simulink model "Bruening_4t_showshuffle"  (R2015a)
settings: Solver=ode4  SolverMode=MultiTasking  StartTime=0.0  StopTime=inf  FixedStep=BKIN_STEP_TIME  RelTol=1e-3
StartFcn:
  |  warndlg('Dexterit-E models cannot run under simulation. Please compile your model and run it from within Dexterit-E.');set_param(bdroot,'SimulationCommand','stop')
model workspace (MAT data in the model file):
  BKIN_STEP_TIME = 0.00025
  col_x = 1
  col_y = 2
  E_TARGET_ON = 3
  E_HOLD_AT_TARGET = 5
  LOGICAL_RADIUS = 4
  START_TARGET_COL = 1
  END_TARGET_COL = 2
  ROTATION_CENTER = 5
  WAIT_AT_1stTARGET_COL = 7
  MAXREACHTIME_COL = 8
  DELAY_POSTTRIAL_COL = 9
  E_STAY_CENTER = 2
  VISUAL_RADIUS = 3
  COLOR = 5
  ALTCOLOR = 6
  STROKECOLOUR = 7
  STROKEWIDTH = 9
  TARGET_EGG = 6
  LABEL_TEXT = 12
  LABEL_COLOUR = 13
  LABEL_HEIGHT = 14
  TEXT_DISPLAY_TARGET = 10
  ALTSTROKECOLOUR = 8
  SEGMENT_COUNT = 11
  E_TARGET_MISS = 6
  END_X = 10
  END_Y = 11
  E_LEFT_RING = 4
  E_START_BLOCK = 10
  BKIN_KINEMATIC_FRAME_SIZE = 400
  E_NO_EVENT = 1
  TARGET_IN_USE = 3
  R_PROB = 4
  E_R_TARG1 = 7
  E_M_TARG1 = 12
  E_R_TARG2 = 8
  E_M_TARG2 = 13
  E_R_TARG3 = 9
  E_M_TARG3 = 14
  E_R_TARG4 = 11
  E_M_TARG4 = 15
  WAIT_TIME = 12
  TONE_DURATION = 13
  FLASH_INTER = 14
  FLASH_NUM = 15
  BREAK_T1 = 16
  BREAK_T2 = 17
  ALTVISUAL_RADIUS = 15
  ALTCOLOR2 = 16
undefined symbols (not defined in the file or in its folder): slselsubs
libraries: Video x15, simulink x12, xpcrtudplib x12, xpcutilitieslib x10, xpcobsoletelib x8, ethercat x2, General x2, slrtlib x2, KINARM_general x1
(part 3 of 6)

== system Bruening_4t_showshuffle/DataLogging/Poll Force Plates/plate1 ==
  gain : Inport
  calib_matrix : Inport  Port=2
  ain_slope : Inport  Port=3
  ain_offset : Inport  Port=4
  orientation : Inport  Port=5
  zero_voltage : Inport  Port=6
  Enable : EnablePort
  Receive : xpcrtudplib/Legacy UDP/Receive   ipAddress=192.168.0.101  ipPort=53795  width=64  vblLen=off  sampletime=BKIN_STEP_TIME
  Terminator : Terminator
  parse packet 1 : MATLAB Function  TreatAsAtomicUnit=on
  Forces P1 : Outport
  Moments P1 : Outport  Port=2
  Timer P1 : Outport  Port=3
  wires:
  parse packet 1/3(timer) -> Timer P1/1
  Receive/2 -> Terminator/1
  gain/1 -> parse packet 1/3(gain)
  Receive/1 -> parse packet 1/1(packet)
  calib_matrix/1 -> parse packet 1/2(calibration)
  parse packet 1/1(forces) -> Forces P1/1
  parse packet 1/2(moments) -> Moments P1/1
  ain_offset/1 -> parse packet 1/5(ain_offset)
  ain_slope/1 -> parse packet 1/4(ain_slope)
  orientation/1 -> parse packet 1/6(orientation)
  zero_voltage/1 -> parse packet 1/7(zero_voltage)

== system Bruening_4t_showshuffle/DataLogging/Poll Force Plates/plate2 ==
  gain : Inport
  calib_matrix : Inport  Port=2
  ain_slope : Inport  Port=3
  ain_offset : Inport  Port=4
  orientation : Inport  Port=5
  zero_voltage : Inport  Port=6
  Enable : EnablePort
  Receive1 : xpcrtudplib/Legacy UDP/Receive   ipAddress=192.168.0.102  ipPort=53796  width=64  vblLen=off  sampletime=BKIN_STEP_TIME
  Terminator : Terminator
  parse packet 1 : MATLAB Function  TreatAsAtomicUnit=on
  Forces P1 : Outport
  Moments P1 : Outport  Port=2
  Timer P1 : Outport  Port=3
  wires:
  parse packet 1/3(timer) -> Timer P1/1
  Receive1/2 -> Terminator/1
  gain/1 -> parse packet 1/3(gain)
  Receive1/1 -> parse packet 1/1(packet)
  calib_matrix/1 -> parse packet 1/2(calibration)
  parse packet 1/1(forces) -> Forces P1/1
  parse packet 1/2(moments) -> Moments P1/1
  ain_offset/1 -> parse packet 1/5(ain_offset)
  ain_slope/1 -> parse packet 1/4(ain_slope)
  orientation/1 -> parse packet 1/6(orientation)
  zero_voltage/1 -> parse packet 1/7(zero_voltage)

== system Bruening_4t_showshuffle/DataLogging/Poll Force Plates/send poll 1 ==
  send packet : Inport
  Enable : EnablePort
  Send : xpcrtudplib/Legacy UDP/Send   ipAddress=192.168.0.101  ipPort=52360  localPort=53795  vblLen=off  sampletime=0.0005
  wires:
  send packet/1 -> Send/1

== system Bruening_4t_showshuffle/DataLogging/Poll Force Plates/send poll 2 ==
  send packet : Inport
  Enable : EnablePort
  Send1 : xpcrtudplib/Legacy UDP/Send   ipAddress=192.168.0.102  ipPort=52360  localPort=53796  vblLen=off  sampletime=0.0005
  wires:
  send packet/1 -> Send1/1

== system Bruening_4t_showshuffle/DataLogging/Poll KINARM/Force Sensor Control ==
  note: This subsystem receives data from force sensors in the KINARM setup, and starts and stops the data transfer in response to changes in
      | the force sensor parameters in the system above. Each KINARM EP can have a force sensor, so there can currently be up to two in a
      | given setup. The force sensors transmit data over UDP, and parameters of the data transfer (such as the data rate and IP address) are
      | configured for each force sensor individually via a web interface they provide. BKIN preconfigures force sensors with IP addresses
      | 192.168.0.10-11, where the first address is given to the sensor for robot 1 and the second to that for robot 2.
  note: Each subsystem also handles the receiving of data from its particular sensor. When a sensor is indicated as present, the latest data from
      | its IP is unpacked and placed into a 1x6 array (zeros are explicitly specified when a sensor is indicated as not present). The arrays for
      | the individual sensors are combined into a 2x6 matrix, similar to how robot data is handled in the system above.
      |
      | Each packet received from a force sensor contains the following:
      |      sequence number [uint32]
      |      internal sequence number [uint32]
      |      system status code [uint32]
      |      x-axis force [int32]
      |      y-axis force [int32]
      |      z-axis force [int32]
      |      x-axis torque [int32]
      |      y-axis torque [int32]
      |      z-axis torque [int32]
      |
      | For more information, again see the ATI Net Interface guide.
  note: Each "force sensor x" subsystem here starts and stops the data transfer from its respective force sensor. When the input flag indicating
      | the presence (1: yes, 0: no) of a force sensor changes, the respective subsystem sends a command message via UDP to that force
      | sensor's IP address that starts or stops the data transfer accordingly. For details about the structure of the command message, see the
      | ATI Net Interface guide.
      |
      | Note that the default setting for all force sensors is 1, for "present", in the system above. This is done so that whenever BKIN's client
      | software applies hardware settings to a task program, it must first lower all force sensor flags and then raise those for whichever sensors
      | are present again. This forces all sensors off in case they were not stopped properly by a previous task. This would not stop data that
      | had been transmitted from being received, so when a force sensor is marked as not present the data is zeroed explicitly.
  has FT : Inport
  Data Type Conversion5 : DataTypeConversion
  Demux : Demux  Outputs=2
  Force Sensor 1 Subsystem : Subsystem
  Force Sensor 2 Subsystem : Subsystem
  Mux8 : Mux  Inputs=2
  Force Sensor Data : Outport
  wires:
  Force Sensor 1 Subsystem/1(Out1) -> Mux8/1
  Force Sensor 2 Subsystem/1(Out1) -> Mux8/2
  Mux8/1 -> Data Type Conversion5/1
  has FT/1 -> Demux/1
  Demux/1 -> Force Sensor 1 Subsystem/1(Force Sensor 1 Present)
  Demux/2 -> Force Sensor 2 Subsystem/1(Force Sensor 2 Present)
  Data Type Conversion5/1 -> Force Sensor Data/1

== system Bruening_4t_showshuffle/DataLogging/Poll KINARM/PMAC Subsystem ==
  note: 1) replaced the variable 'orientation' with two variables: 'robot_orientation' and 'arm_orientation'.  Add comments to better explain.
      | 2) replaced the variables 'uncorrected_shoulder_angle' and 'uncorrected_elbow_angle' with 'relative_shoulder_angle' and 'relative_elbow_angle'
      | 3) replaced the variables corrected_shoulder_angle and corrected_elbow_angle with shoulder_angle and elbow_angle
      | 4) primary encoder data was not being corrected properly (for errors in non-perfect parallelogram structure) in the original.  This has now been fixed.
      | 5) replaced "if (robot_type < 1.0 && orientation == 2) || (robot_type > 0.0 && orientation == 1)"
      |             with "(robot_orientation == -1)"
  note: This block provides access to KINARM data for both BKIN client software and task program authors. Client software must provide
      | correct hardware information and calibration parameters for each KINARM, and this information is subsequently used to read
      | and scale data from the motion control card. The KINARM data and other attributes of the KINARM setup controlled by client
      | software, such as which arm is "dominant" for the KINARM EXO or EP, are combined into the KINdata structure. Arm kinematics
      | are output for inclusion in the current data frame.
      |
      | This block also offers client software access to the motion control card DPRAM via the DPRAM access subsystem.
      |
      | Note: The mask replaces the ZeroTorque constant with a From block that includes the commanded torques providing the model
      | includes an instance of the load-applying block.
      |
      | Note: For each Goto block created here, a corresponding From block is included in the Terminators for Gotos subsystem. This is
      | solely to prevent unnecessary warnings at the Matlab prompt if such From blocks are not present.
  enable : Inport
  run : Inport  Port=2
  pmac robot params : Inport  Port=3
  Bus Selector : BusSelector  OutputSignals=pmac robot1 params,pmac robot2 params
  read_pmac : Subsystem
      settings: RTWSystemCode=Nonreusable function  RTWFileNameOpts=Use function name
  update settings : Subsystem
  pmac force scale : Outport
  wires:
  read_pmac/1(robot data) -> update settings/1(Kinematics)
  read_pmac/2(servo counter) -> update settings/2(Servo counter)
  read_pmac/3(delay estimates) -> update settings/3(delay estimates)
  read_pmac/4(primary_encoder data) -> update settings/4(primry enc data)
  read_pmac/5(ep calibration bitfield) -> update settings/5(EP Calibration Button)
  read_pmac/6(status data) -> update settings/6(Robot status)
  run/1 -> update settings/Trigger
  enable/1 -> [enable]
  [enable] -> read_pmac/Enable
  pmac robot params/1 -> Bus Selector/1
  Bus Selector/1 -> read_pmac/1(pmac robot1 params)  "<pmac robot1 params>"
  Bus Selector/2 -> read_pmac/2(pmac robot2 params)  "<pmac robot2 params>"
  read_pmac/7(force scale) -> pmac force scale/1

== system Bruening_4t_showshuffle/DataLogging/Poll KINARM/constants ==
  Bus Creator : BusCreator
  Bus Creator1 : BusCreator
  Bus Creator2 : BusCreator  Inputs=2
  arm1 : Subsystem
  arm2 : Subsystem
  update constants : Constant
  update constants subsystem : Subsystem
  pmac motor params : Outport
  calibrations : Outport  Port=2
  wires:
  arm1/2(pmac motor params) -> Bus Creator1/1  "pmac robot1 params"
  arm2/2(pmac motor params) -> Bus Creator1/2  "pmac robot2 params"
  arm1/4(motor parameters) -> Bus Creator1/3  "robot1MotorParams"
  arm2/4(motor parameters) -> Bus Creator1/4  "robot2MotorParams"
  arm1/3(hardware settings) -> Bus Creator/2  "robot1 hardware settings"
  arm2/3(hardware settings) -> Bus Creator/4  "robot2 hardware settings"
  Bus Creator/1 -> update constants subsystem/1(Params)
  update constants/1 -> update constants subsystem/Enable
  arm1/1(calibration) -> Bus Creator/1, Bus Creator2/1  "robot1 calibration params"
  arm2/1(calibration) -> Bus Creator/3, Bus Creator2/2  "robot2 calibration params"
  Bus Creator1/1 -> pmac motor params/1  "motor params"
  Bus Creator2/1 -> calibrations/1

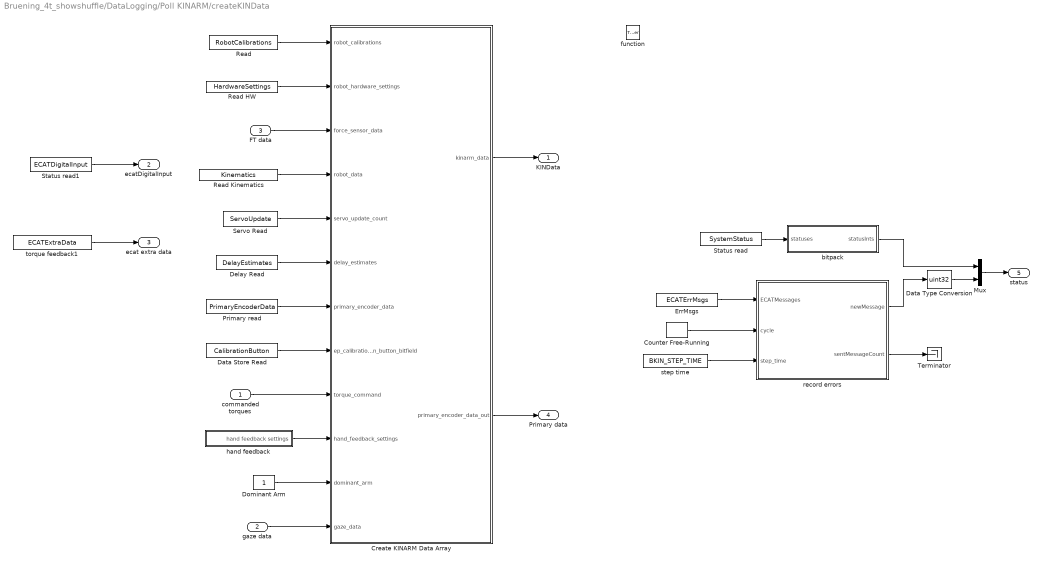
== system Bruening_4t_showshuffle/DataLogging/Poll KINARM/createKINData ==
  commanded torques : Inport
  gaze data : Inport  Port=2
  FT data : Inport  Port=3
  function : TriggerPort  TriggerType=function-call
  Counter Free-Running : simulink/Sources/Counter Free-Running  NumBits=32  tsamp=-1
  Create KINARM Data Array : MATLAB Function  TreatAsAtomicUnit=on
  Data Store Read : DataStoreRead  DataStoreName=CalibrationButton
  Data Type Conversion : DataTypeConversion  OutDataTypeStr=uint32
  Delay Read : DataStoreRead  DataStoreName=DelayEstimates
  Dominant Arm : Constant
  ErrMsgs : DataStoreRead  DataStoreName=ECATErrMsgs
  Mux : Mux  Inputs=2
  Primary read : DataStoreRead  DataStoreName=PrimaryEncoderData
  Read : DataStoreRead  DataStoreName=RobotCalibrations
  Read HW : DataStoreRead  DataStoreName=HardwareSettings
  Read Kinematics : DataStoreRead  DataStoreName=Kinematics
  Servo Read : DataStoreRead  DataStoreName=ServoUpdate
  Status read : DataStoreRead  DataStoreName=SystemStatus
  Status read1 : DataStoreRead  DataStoreName=ECATDigitalInput
  Terminator : Terminator
  bitpack : MATLAB Function  TreatAsAtomicUnit=on
  hand feedback : Subsystem
  record errors : MATLAB Function  TreatAsAtomicUnit=on
  step time : Constant  Value=BKIN_STEP_TIME
  torque feedback1 : DataStoreRead  DataStoreName=ECATExtraData
  KINData : Outport
  ecatDigitalInput : Outport  Port=2
  ecat extra data : Outport  Port=3
  Primary data : Outport  Port=4
  status : Outport  Port=5
  wires:
  hand feedback/1(hand feedback settings) -> Create KINARM Data Array/10(hand_feedback_settings)
  Read/1 -> Create KINARM Data Array/1(robot_calibrations)
  Servo Read/1 -> Create KINARM Data Array/5(servo_update_count)
  Data Store Read/1 -> Create KINARM Data Array/8(ep_calibration_button_bitfield)
  Dominant Arm/1 -> Create KINARM Data Array/11(dominant_arm)
  Delay Read/1 -> Create KINARM Data Array/6(delay_estimates)
  Read Kinematics/1 -> Create KINARM Data Array/4(robot_data)
  Primary read/1 -> Create KINARM Data Array/7(primary_encoder_data)
  Read HW/1 -> Create KINARM Data Array/2(robot_hardware_settings)
  gaze data/1 -> Create KINARM Data Array/12(gaze_data)
  Create KINARM Data Array/2(primary_encoder_data_out) -> Primary data/1
  FT data/1 -> Create KINARM Data Array/3(force_sensor_data)
  Create KINARM Data Array/1(kinarm_data) -> KINData/1
  commanded torques/1 -> Create KINARM Data Array/9(torque_command)
  Status read1/1 -> ecatDigitalInput/1
  torque feedback1/1 -> ecat extra data/1
  ErrMsgs/1 -> record errors/1(ECATMessages)
  Status read/1 -> bitpack/1(statuses)
  record errors/1(newMessage) -> Data Type Conversion/1
  Mux/1 -> status/1
  Data Type Conversion/1 -> Mux/2
  Counter Free-Running/1 -> record errors/2(cycle)
  step time/1 -> record errors/3(step_time)
  record errors/2(sentMessageCount) -> Terminator/1
  bitpack/1(statusInts) -> Mux/1

== system Bruening_4t_showshuffle/DataLogging/Poll KINARM/make KINData bus ==
  KINData : Inport
  ECAT Digital Input : Inport  Port=2
  ecat recorded torques : Inport  Port=3
  Bus Creator1 : BusCreator  Inputs=26
  Bus Creator2 : BusCreator  Inputs=26
  Bus Creator3 : BusCreator  Inputs=6
  Bus Creator4 : BusCreator
  Bus Creator5 : BusCreator  Inputs=5
  Bus Creator6 : BusCreator  Inputs=6
  Selector : Selector  NumberOfDimensions=2  InputPortWidth=3  IndexOptions=Index vector (dialog),Select all  Indices=[1],1  OutputSizes=1,1
  Selector1 : Selector  NumberOfDimensions=2  InputPortWidth=3  IndexOptions=Index vector (dialog),Select all  Indices=[2],1  OutputSizes=1,1
  Selector2 : Selector  NumberOfDimensions=2  InputPortWidth=3  IndexOptions=Index vector (dialog),Select all  Indices=[3],1  OutputSizes=1,1
  Selector3 : Selector  Indices=[1 2]
  Selector4 : Selector  Indices=[3, 4]
  Selector5 : Selector  Indices=[5 6]
  Selector6 : Selector  Indices=[7, 8]
  splitKINData arm1 : MATLAB Function  TreatAsAtomicUnit=on
  splitKINData arm2 : MATLAB Function  TreatAsAtomicUnit=on
  splitKINDataGeneral : MATLAB Function  TreatAsAtomicUnit=on
  KINData_bus : Outport
  wires:
  splitKINDataGeneral/10(hasGaze) -> Bus Creator3/1  "has_gaze"
  splitKINDataGeneral/11(gazeFB) -> Bus Creator3/2  "gazeFB_control"
  splitKINDataGeneral/12(gazeLocation) -> Bus Creator3/3  "gaze_location"
  splitKINDataGeneral/13(gazeTimestamp) -> Bus Creator3/4  "gaze_timestamp"
  splitKINDataGeneral/14(gazePupilArea) -> Bus Creator3/5  "gaze_pupil_area"
  splitKINDataGeneral/15(gazeEvent) -> Bus Creator3/6  "gaze_event"
  splitKINData arm1/1(link_lengths) -> Bus Creator1/1  "a1_link_lengths"
  splitKINData arm1/2(pointer_offset) -> Bus Creator1/2  "a1_pointer_offset"
  splitKINData arm1/3(shoulder_loc) -> Bus Creator1/3  "a1_shoulder_location"
  splitKINData arm1/4(arm_orientation) -> Bus Creator1/4  "a1_arm_orientation"
  splitKINData arm1/5(shoulder_ang) -> Bus Creator1/5  "a1_shoulder_angle"
  splitKINData arm1/6(elbow_ang) -> Bus Creator1/6  "a1_elbow_angle"
  splitKINData arm1/7(shoulder_velocity) -> Bus Creator1/7  "a1_shoulder_velocity"
  splitKINData arm1/8(elbow_velocity) -> Bus Creator1/8  "a1_elbow_velocity"
  splitKINData arm1/9(shoulder_acceleration) -> Bus Creator1/9  "a1_shoulder_acceleration"
  splitKINData arm1/10(elbow_acceleration) -> Bus Creator1/10  "a1_elbow_acceleration"
  splitKINData arm1/11(joint_torque_cmd) -> Bus Creator1/11  "a1_joint_torque_command"
  splitKINData arm1/12(motor_torque_cmd) -> Bus Creator1/12  "a1_motor_torque_command"
  splitKINData arm1/13(link_angle) -> Bus Creator1/13  "a1_link_angles"
  splitKINData arm1/14(link_velocity) -> Bus Creator1/14  "a1_link_velocities"
  splitKINData arm1/15(link_acceleration) -> Bus Creator1/15  "a1_link_accelerations"
  splitKINData arm1/16(hand_position) -> Bus Creator1/16  "a1_hand_position"
  splitKINData arm1/17(hand_velocity) -> Bus Creator1/17  "a1_hand_velocities"
  splitKINData arm1/18(hand_acceleration) -> Bus Creator1/18  "a1_hand_accelerations"
  splitKINData arm1/19(motor_status) -> Bus Creator1/19  "a1_motor_status"
  splitKINData arm1/20(force_sensor_force_uvw) -> Bus Creator1/20  "a1_force_sensor_force_uvw"
  splitKINData arm1/21(force_sensor_torque_uvw) -> Bus Creator1/21  "a1_force_sensor_torque_uvw"
  splitKINData arm1/22(force_sensor_force_xyz) -> Bus Creator1/22  "a1_force_sensor_force_xyz"
  splitKINData arm1/23(force_sensor_torque_xyz) -> Bus Creator1/23  "a1_force_sensor_torque_xyz"
  splitKINData arm1/24(force_sensor_timestamp) -> Bus Creator1/24  "a1_force_sensor_timestamp"
  splitKINData arm2/1(link_lengths) -> Bus Creator2/1  "a2_link_lengths"
  splitKINData arm2/2(pointer_offset) -> Bus Creator2/2  "a2_pointer_offset"
  splitKINData arm2/3(shoulder_loc) -> Bus Creator2/3  "a2_shoulder_location"
  splitKINData arm2/4(arm_orientation) -> Bus Creator2/4  "a2_arm_orientation"
  splitKINData arm2/5(shoulder_ang) -> Bus Creator2/5  "a2_shoulder_angle"
  splitKINData arm2/6(elbow_ang) -> Bus Creator2/6  "a2_elbow_angle"
  splitKINData arm2/7(shoulder_velocity) -> Bus Creator2/7  "a2_shoulder_velocity"
  splitKINData arm2/8(elbow_velocity) -> Bus Creator2/8  "a2_elbow_velocity"
  splitKINData arm2/9(shoulder_acceleration) -> Bus Creator2/9  "a2_shoulder_acceleration"
  splitKINData arm2/10(elbow_acceleration) -> Bus Creator2/10  "a2_elbow_acceleration"
  splitKINData arm2/11(joint_torque_cmd) -> Bus Creator2/11  "a2_joint_torque_command"
  splitKINData arm2/12(motor_torque_cmd) -> Bus Creator2/12  "a2_motor_torque_command"
  splitKINData arm2/13(link_angle) -> Bus Creator2/13  "a2_link_angles"
  splitKINData arm2/14(link_velocity) -> Bus Creator2/14  "a2_link_velocities"
  splitKINData arm2/15(link_acceleration) -> Bus Creator2/15  "a2_link_accelerations"
  splitKINData arm2/16(hand_position) -> Bus Creator2/16  "a2_hand_position"
  splitKINData arm2/17(hand_velocity) -> Bus Creator2/17  "a2_hand_velocities"
  splitKINData arm2/18(hand_acceleration) -> Bus Creator2/18  "a2_hand_accelerations"
  splitKINData arm2/19(motor_status) -> Bus Creator2/19  "a2_motor_status"
  splitKINData arm2/20(force_sensor_force_uvw) -> Bus Creator2/20  "a2_force_sensor_force_uvw"
  splitKINData arm2/21(force_sensor_torque_uvw) -> Bus Creator2/21  "a2_force_sensor_torque_uvw"
  splitKINData arm2/22(force_sensor_force_xyz) -> Bus Creator2/22  "a2_force_sensor_force_xyz"
  splitKINData arm2/23(force_sensor_torque_xyz) -> Bus Creator2/23  "a2_force_sensor_torque_xyz"
  splitKINData arm2/24(force_sensor_timestamp) -> Bus Creator2/24  "a2_force_sensor_timestamp"
  Selector/1 -> splitKINData arm1/1(robot_row)
  Selector1/1 -> splitKINData arm2/1(robot_row)
  splitKINDataGeneral/1(active_arm) -> Bus Creator4/1  "active_arm"
  splitKINDataGeneral/2(delayEstimates) -> Bus Creator4/2  "delay_estimates"
  splitKINDataGeneral/3(servoCounter) -> Bus Creator4/3  "servo_counter"
  splitKINDataGeneral/4(calibrationButtonBits) -> Bus Creator4/4  "calibration_button_bits"
  splitKINDataGeneral/5(handFF) -> Bus Creator5/1  "handFB_feed_forward_time"
  splitKINDataGeneral/6(handFBArm) -> Bus Creator5/2  "handFB_arm"
  splitKINDataGeneral/7(handFBRadius) -> Bus Creator5/3  "handFB_radius"
  splitKINDataGeneral/8(handFBControl) -> Bus Creator5/4  "handFB_control"
  splitKINDataGeneral/9(handFBColor) -> Bus Creator5/5  "handFB_color"
  Bus Creator4/1 -> Bus Creator6/1  "KINDataGeneral"
  Bus Creator5/1 -> Bus Creator6/2  "Hand_feedback"
  Bus Creator3/1 -> Bus Creator6/3  "gaze"
  Bus Creator1/1 -> Bus Creator6/4  "Robot1"
  Bus Creator2/1 -> Bus Creator6/5  "Robot2"
  KINData/1 -> Selector1/1, Selector/1, Selector2/1
  Bus Creator6/1 -> KINData_bus/1
  Selector2/1 -> splitKINDataGeneral/1(kinarm_data)
  ECAT Digital Input/1 -> Bus Creator6/6  "ECAT Digital Input"
  ecat recorded torques/1 -> Selector3/1, Selector5/1, Selector4/1, Selector6/1
  Selector3/1 -> Bus Creator1/25  "a1_ecatRecordedMotorTorques"
  Selector4/1 -> Bus Creator2/25  "a2_ecatRecordedMotorTorques"
  Selector5/1 -> Bus Creator1/26  "a1_ecatCurrentLimitEnabled"
  Selector6/1 -> Bus Creator2/26  "a2_ecatCurrentLimitEnabled"

== system Bruening_4t_showshuffle/DataLogging/Poll KINARM/split_primary ==
  primary data : Inport
  Bus Creator1 : BusCreator  Inputs=3
  Bus Creator2 : BusCreator  Inputs=2
  Bus Creator4 : BusCreator  Inputs=3
  Selector1 : Selector  NumberOfDimensions=2  InputPortWidth=3  IndexOptions=Index vector (dialog),Select all  Indices=[2],1  OutputSizes=1,1
  Selector2 : Selector  NumberOfDimensions=2  InputPortWidth=3  IndexOptions=Index vector (dialog),Select all  Indices=[1],1  OutputSizes=1,1
  split_primary : MATLAB Function  TreatAsAtomicUnit=on
  split_primary1 : MATLAB Function  TreatAsAtomicUnit=on
  primary_data_bus : Outport
  wires:
  split_primary/1(link_angles) -> Bus Creator4/1  "a1_link_angles"
  split_primary/2(link_velocities) -> Bus Creator4/2  "a1_link_velocities"
  split_primary/3(link_acceleration) -> Bus Creator4/3  "a1_link_accelerations"
  primary data/1 -> Selector2/1, Selector1/1
  Selector2/1 -> split_primary/1(primary_data)
  split_primary1/1(link_angles) -> Bus Creator1/1  "a2_link_angles"
  split_primary1/2(link_velocities) -> Bus Creator1/2  "a2_link_velocities"
  split_primary1/3(link_acceleration) -> Bus Creator1/3  "a2_link_accelerations"
  Selector1/1 -> split_primary1/1(primary_data)
  Bus Creator4/1 -> Bus Creator2/1  "robot1"
  Bus Creator1/1 -> Bus Creator2/2  "robot2"
  Bus Creator2/1 -> primary_data_bus/1

== system Bruening_4t_showshuffle/DataLogging/apply loads/apply pmac loads ==
  Force scale : Inport
  Torques : Inport  Port=2
  Robot 1 motor parms : Inport  Port=3
  Robot 2 motor parms : Inport  Port=4
  Enable : EnablePort
  Bus Selector : BusSelector  OutputSignals=R1.Arm Orientation,R1.M1 orientation,R1.M2 Orientation,R1.M1 Gear Ratio,R1.M2 Gear Ratio,torque constant  OutputAsBus=on
  Bus Selector1 : BusSelector  OutputSignals=R2.Arm Orientation,R2.M1 orientation,R2.M2 Orientation,R2.M1 Gear Ratio,R2.M2 Gear Ratio,torque constant  OutputAsBus=on
  Bus to Vector : BusToVector
  Bus to Vector1 : BusToVector
  Data Type Conversion : DataTypeConversion
  Data Type Conversion1 : DataTypeConversion
  Data Type Conversion6 : DataTypeConversion  OutDataTypeStr=single
  Product : Product  RndMeth=Zero
  S-Function1 : S-Function  FunctionName=mcc_apply_loads
  wires:
  Torques/1 -> Product/1
  Data Type Conversion6/1 -> S-Function1/1
  Product/1 -> Data Type Conversion6/1
  Bus to Vector1/1 -> Data Type Conversion1/1
  Bus to Vector/1 -> Data Type Conversion/1
  Force scale/1 -> Product/2
  Robot 2 motor parms/1 -> Bus Selector1/1
  Data Type Conversion/1 -> S-Function1/2
  Data Type Conversion1/1 -> S-Function1/3
  Robot 1 motor parms/1 -> Bus Selector/1
  Bus Selector/1 -> Bus to Vector/1
  Bus Selector1/1 -> Bus to Vector1/1

== system Bruening_4t_showshuffle/DataLogging/Network Transfer Subsystem/Data Packing Subsystem/Counter ==
  Constant : Constant
  Sum : Sum  Inputs=|++  SaturateOnIntegerOverflow=on
  Unit Delay : UnitDelay  SampleTime=-1
  Y : Outport
  wires:
  Constant/1 -> Sum/2
  Sum/1 -> Unit Delay/1, Y/1
  Unit Delay/1 -> Sum/1

== system Bruening_4t_showshuffle/DataLogging/Poll KINARM/Force Sensor Control/Force Sensor 1 Subsystem ==
  Force Sensor 1 Present : Inport
  Byte Reversal : xpcutilitieslib/Byte Reversal   numInp=1
  Byte Reversal1 : xpcutilitieslib/Byte Reversal   numInp=1
  Constant : Constant  Value=zeros(1, 7);  OutDataTypeStr=double
  Create timestamp : MATLAB Function  TreatAsAtomicUnit=on
  Data Type Conversion : DataTypeConversion
  Detect Change : simulink/Logic and Bit Operations/Detect Change  vinit=-1  InputProcessing=Inherited  OutDataTypeStr=uint8
  If Action Subsystem : Subsystem  TreatAsAtomicUnit=on
  Mux : Mux  Inputs=2
  Receive from Robot 1 Force Sensor : xpcrtudplib/Legacy UDP/Receive   ipAddress=192.168.0.10  ipPort=51000  width=36  vblLen=off  sampletime=BKIN_STEP_TIME
  Switch : Switch  Criteria=u2 > Threshold
  Terminator : Terminator
  Unpack : xpcobsoletelib/Utilities/Unpack   dimensions={3, 6}  datatypes={'uint32', 'int32'}  byteAlign=1
  Out1 : Outport
  wires:
  Receive from Robot 1 Force Sensor/1 -> Unpack/1
  Receive from Robot 1 Force Sensor/2 -> Terminator/1
  Force Sensor 1 Present/1 -> Switch/2, If Action Subsystem/1(In1), Detect Change/1
  Constant/1 -> Switch/3
  Switch/1 -> Out1/1
  Unpack/2 -> Byte Reversal/1
  Unpack/1 -> Byte Reversal1/1
  Byte Reversal/1 -> Data Type Conversion/1
  Detect Change/1 -> If Action Subsystem/Enable
  Create timestamp/1(timestamp_out) -> Mux/2
  Data Type Conversion/1 -> Mux/1
  Mux/1 -> Switch/1
  Byte Reversal1/1 -> Create timestamp/1(times_in)

== system Bruening_4t_showshuffle/DataLogging/Poll KINARM/Force Sensor Control/Force Sensor 2 Subsystem ==
  Force Sensor 2 Present : Inport
  Byte Reversal : xpcutilitieslib/Byte Reversal   numInp=1
  Byte Reversal1 : xpcutilitieslib/Byte Reversal   numInp=1
  Constant1 : Constant  Value=zeros(1, 7);  OutDataTypeStr=double
  Create timestamp : MATLAB Function  TreatAsAtomicUnit=on
  Data Transfer Start Subsystem : Subsystem  TreatAsAtomicUnit=on
  Data Type Conversion1 : DataTypeConversion
  Detect Change : simulink/Logic and Bit Operations/Detect Change  vinit=-1  InputProcessing=Inherited  OutDataTypeStr=uint8
  Mux : Mux  Inputs=2
  Receive from Robot 2 Force Sensor : xpcrtudplib/Legacy UDP/Receive   ipAddress=192.168.0.11  ipPort=51001  width=36  vblLen=off  sampletime=BKIN_STEP_TIME
  Switch1 : Switch  Criteria=u2 > Threshold
  Terminator1 : Terminator
  Unpack1 : xpcobsoletelib/Utilities/Unpack   dimensions={3, 6}  datatypes={'uint32', 'int32'}  byteAlign=1
  Out1 : Outport
  wires:
  Receive from Robot 2 Force Sensor/1 -> Unpack1/1
  Receive from Robot 2 Force Sensor/2 -> Terminator1/1
  Force Sensor 2 Present/1 -> Data Transfer Start Subsystem/1(In2), Detect Change/1, Switch1/2
  Constant1/1 -> Switch1/3
  Switch1/1 -> Out1/1
  Unpack1/2 -> Byte Reversal/1
  Byte Reversal/1 -> Data Type Conversion1/1
  Detect Change/1 -> Data Transfer Start Subsystem/Enable
  Unpack1/1 -> Byte Reversal1/1
  Data Type Conversion1/1 -> Mux/1
  Create timestamp/1(timestamp_out) -> Mux/2
  Mux/1 -> Switch1/1
  Byte Reversal1/1 -> Create timestamp/1(times_in)

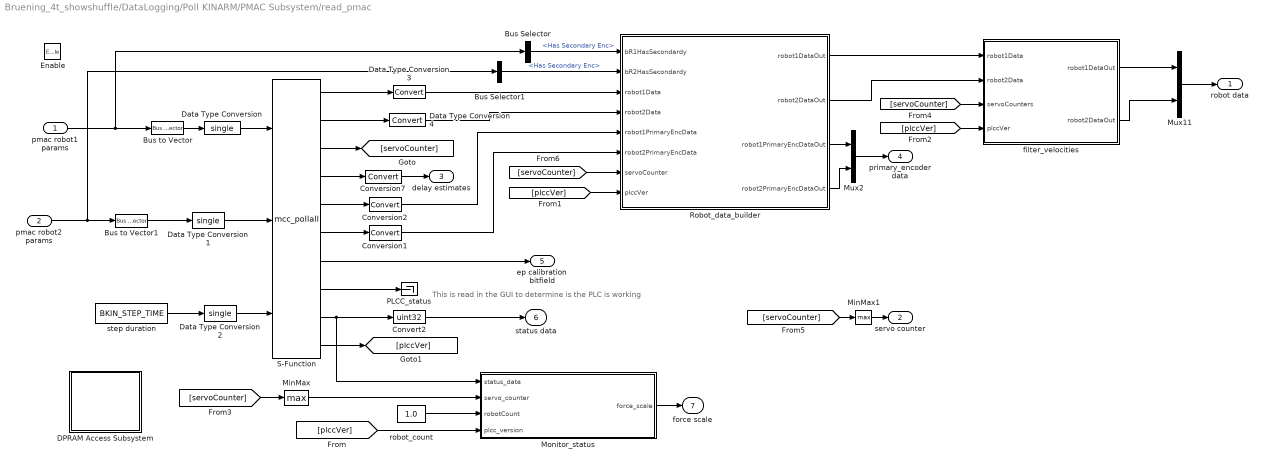
== system Bruening_4t_showshuffle/DataLogging/Poll KINARM/PMAC Subsystem/read_pmac ==
  note: This is read in the GUI to determine is the PLC is working
  pmac robot1 params : Inport
  pmac robot2 params : Inport  Port=2
  Enable : EnablePort
  Bus Selector : BusSelector  OutputSignals=R1.Has Secondary Enc
  Bus Selector1 : BusSelector  OutputSignals=R2.Has Secondary Enc
  Bus to Vector : BusToVector
  Bus to Vector1 : BusToVector
  Conversion1 : DataTypeConversion
  Conversion2 : DataTypeConversion
  Conversion7 : DataTypeConversion
  Convert2 : DataTypeConversion  OutDataTypeStr=uint32
  DPRAM Access Subsystem : Subsystem
  Data Type Conversion : DataTypeConversion  OutDataTypeStr=single
  Data Type Conversion1 : DataTypeConversion  OutDataTypeStr=single
  Data Type Conversion2 : DataTypeConversion  OutDataTypeStr=single
  Data Type Conversion3 : DataTypeConversion
  Data Type Conversion4 : DataTypeConversion
  MinMax : MinMax  Function=max
  MinMax1 : MinMax  Function=max
  Monitor_status : MATLAB Function  TreatAsAtomicUnit=on  SystemSampleTime=BKIN_STEP_TIME
  Mux11 : Mux  Inputs=2
  Mux2 : Mux  Inputs=2
  PLCC_status : Terminator
  Robot_data_builder : MATLAB Function  TreatAsAtomicUnit=on
  S-Function : S-Function  FunctionName=mcc_pollall
  filter_velocities : MATLAB Function  TreatAsAtomicUnit=on
  robot_count : Constant  Value=1.0
  step duration : Constant  Value=BKIN_STEP_TIME  OutDataTypeStr=double
  robot data : Outport
  servo counter : Outport  Port=2
  delay estimates : Outport  Port=3
  primary_encoder data : Outport  Port=4
  ep calibration bitfield : Outport  Port=5
  status data : Outport  Port=6
  force scale : Outport  Port=7
  wires:
  MinMax/1 -> Monitor_status/2(servo_counter)
  pmac robot1 params/1 -> Bus to Vector/1, Bus Selector/1
  pmac robot2 params/1 -> Bus to Vector1/1, Bus Selector1/1
  Mux11/1 -> robot data/1
  Conversion7/1 -> delay estimates/1
  robot_count/1 -> Monitor_status/3(robotCount)
  Data Type Conversion4/1 -> Robot_data_builder/4(robot2Data)
  Data Type Conversion3/1 -> Robot_data_builder/3(robot1Data)
  Robot_data_builder/3(robot1PrimaryEncDataOut) -> Mux2/1
  Robot_data_builder/4(robot2PrimaryEncDataOut) -> Mux2/2
  Mux2/1 -> primary_encoder data/1
  Conversion2/1 -> Robot_data_builder/5(robot1PrimaryEncData)
  Conversion1/1 -> Robot_data_builder/6(robot2PrimaryEncData)
  S-Function/4 -> Conversion7/1
  S-Function/5 -> Conversion2/1
  step duration/1 -> Data Type Conversion2/1
  Data Type Conversion/1 -> S-Function/1
  S-Function/9 -> Monitor_status/1(status_data), Convert2/1
  S-Function/1 -> Data Type Conversion3/1
  Data Type Conversion1/1 -> S-Function/2
  Convert2/1 -> status data/1
  S-Function/8 -> PLCC_status/1
  S-Function/6 -> Conversion1/1
  S-Function/7 -> ep calibration bitfield/1
  S-Function/2 -> Data Type Conversion4/1
  Monitor_status/1(force_scale) -> force scale/1
  Bus to Vector/1 -> Data Type Conversion/1
  Bus to Vector1/1 -> Data Type Conversion1/1
  Bus Selector/1 -> Robot_data_builder/1(bR1HasSecondardy)  "<Has Secondary Enc>"
  Bus Selector1/1 -> Robot_data_builder/2(bR2HasSecondardy)  "<Has Secondary Enc>"
  Data Type Conversion2/1 -> S-Function/3
  Robot_data_builder/1(robot1DataOut) -> filter_velocities/1(robot1Data)
  Robot_data_builder/2(robot2DataOut) -> filter_velocities/2(robot2Data)
  S-Function/3 -> [servoCounter]
  S-Function/10 -> [plccVer]
  [plccVer] -> Monitor_status/4(plcc_version)
  [plccVer] -> Robot_data_builder/8(plccVer)
  [plccVer] -> filter_velocities/4(plccVer)
  [servoCounter] -> MinMax/1
  [servoCounter] -> filter_velocities/3(servoCounters)
  filter_velocities/1(robot1DataOut) -> Mux11/1
  filter_velocities/2(robot2DataOut) -> Mux11/2
  [servoCounter] -> MinMax1/1
  [servoCounter] -> Robot_data_builder/7(servoCounter)
  MinMax1/1 -> servo counter/1

== system Bruening_4t_showshuffle/DataLogging/Poll KINARM/PMAC Subsystem/update settings ==
  Kinematics : Inport
  Servo counter : Inport  Port=2
  delay estimates : Inport  Port=3
  primry enc data : Inport  Port=4
  EP Calibration Button : Inport  Port=5
  Robot status : Inport  Port=6
  function : TriggerPort  TriggerType=function-call
  Data Store Write1 : DataStoreWrite  DataStoreName=Kinematics
  Data Store Write2 : DataStoreWrite  DataStoreName=ServoUpdate
  Data Store Write3 : DataStoreWrite  DataStoreName=DelayEstimates
  Data Store Write4 : DataStoreWrite  DataStoreName=PrimaryEncoderData
  Data Store Write5 : DataStoreWrite  DataStoreName=CalibrationButton
  Data Store Write7 : DataStoreWrite  DataStoreName=SystemStatus
  update status format : MATLAB Function  TreatAsAtomicUnit=on
  wires:
  Kinematics/1 -> Data Store Write1/1
  Servo counter/1 -> Data Store Write2/1
  delay estimates/1 -> Data Store Write3/1
  primry enc data/1 -> Data Store Write4/1
  EP Calibration Button/1 -> Data Store Write5/1
  update status format/1(outStatus) -> Data Store Write7/1
  Robot status/1 -> update status format/1(pmacStatus)

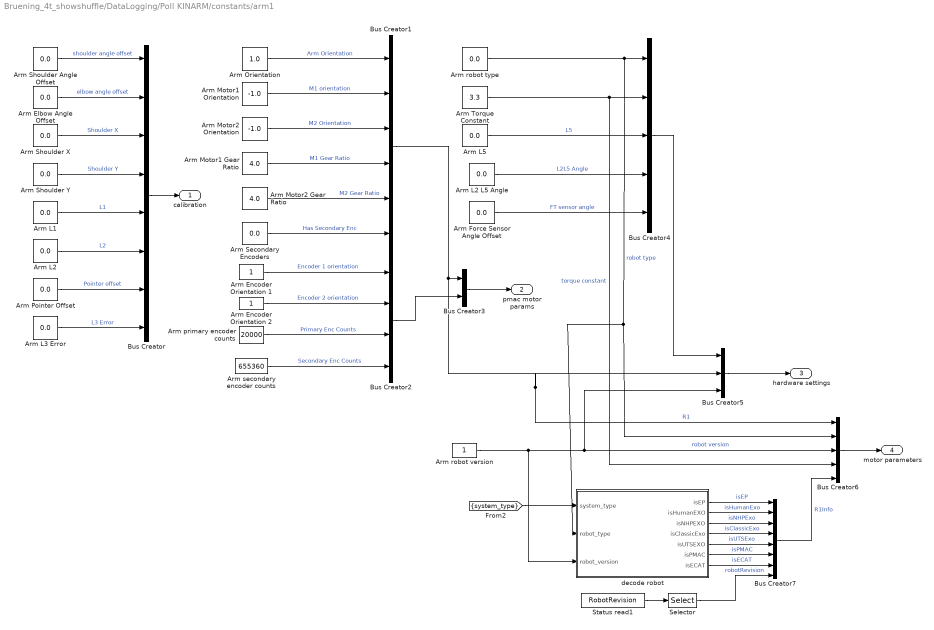
== system Bruening_4t_showshuffle/DataLogging/Poll KINARM/constants/arm1 ==
  Arm Elbow Angle Offset : Constant  Value=0.0  SampleTime=BKIN_STEP_TIME
  Arm Encoder Orientation 1 : Constant
  Arm Encoder Orientation 2 : Constant
  Arm Force Sensor Angle Offset : Constant  Value=0.0
  Arm L1 : Constant  Value=0.0  SampleTime=BKIN_STEP_TIME
  Arm L2 : Constant  Value=0.0  SampleTime=BKIN_STEP_TIME
  Arm L2 L5 Angle : Constant  Value=0.0
  Arm L3 Error : Constant  Value=0.0  SampleTime=BKIN_STEP_TIME
  Arm L5 : Constant  Value=0.0
  Arm Motor1 Gear Ratio : Constant  Value=4.0
  Arm Motor1 Orientation : Constant  Value=-1.0
  Arm Motor2 Gear Ratio : Constant  Value=4.0
  Arm Motor2 Orientation : Constant  Value=-1.0
  Arm Orientation : Constant  Value=1.0
  Arm Pointer Offset : Constant  Value=0.0  SampleTime=BKIN_STEP_TIME
  Arm Secondary Encoders : Constant  Value=0.0
  Arm Shoulder Angle Offset : Constant  Value=0.0  SampleTime=BKIN_STEP_TIME
  Arm Shoulder X : Constant  Value=0.0  SampleTime=BKIN_STEP_TIME
  Arm Shoulder Y : Constant  Value=0.0  SampleTime=BKIN_STEP_TIME
  Arm Torque Constant : Constant  Value=3.3
  Arm primary encoder counts : Constant  Value=20000
  Arm robot type : Constant  Value=0.0
  Arm robot version : Constant
  Arm secondary encoder counts : Constant  Value=655360
  Bus Creator : BusCreator  Inputs=8
  Bus Creator1 : BusCreator  Inputs=6
  Bus Creator2 : BusCreator
  Bus Creator3 : BusCreator  Inputs=2
  Bus Creator4 : BusCreator  Inputs=5
  Bus Creator5 : BusCreator  Inputs=3
  Bus Creator6 : BusCreator  Inputs=5
  Bus Creator7 : BusCreator  Inputs=8
  Selector : Selector  Indices=[1]
  Status read1 : DataStoreRead  DataStoreName=RobotRevision
  decode robot : MATLAB Function  TreatAsAtomicUnit=on
  calibration : Outport
  pmac motor params : Outport  Port=2
  hardware settings : Outport  Port=3
  motor parameters : Outport  Port=4
  wires:
  Arm secondary encoder counts/1 -> Bus Creator2/4  "Secondary Enc Counts"
  Arm primary encoder counts/1 -> Bus Creator2/3  "Primary Enc Counts"
  Arm Orientation/1 -> Bus Creator1/1  "Arm Orientation"
  Arm Motor1 Orientation/1 -> Bus Creator1/2  "M1 orientation"
  Arm Motor2 Orientation/1 -> Bus Creator1/3  "M2 Orientation"
  Arm Motor1 Gear Ratio/1 -> Bus Creator1/4  "M1 Gear Ratio"
  Arm Motor2 Gear Ratio/1 -> Bus Creator1/5  "M2 Gear Ratio"
  Arm Secondary Encoders/1 -> Bus Creator1/6  "Has Secondary Enc"
  Arm robot type/1 -> Bus Creator4/1, Bus Creator6/2, decode robot/2(robot_type)  "robot type"
  Arm Torque Constant/1 -> Bus Creator4/2, Bus Creator6/4  "torque constant"
  Arm L5/1 -> Bus Creator4/3  "L5"
  Arm L2 L5 Angle/1 -> Bus Creator4/4  "L2L5 Angle"
  Bus Creator4/1 -> Bus Creator5/1
  Arm Force Sensor Angle Offset/1 -> Bus Creator4/5  "FT sensor angle"
  Arm Encoder Orientation 1/1 -> Bus Creator2/1  "Encoder 1 orientation"
  Arm Encoder Orientation 2/1 -> Bus Creator2/2  "Encoder 2 orientation"
  Bus Creator2/1 -> Bus Creator3/2
  Bus Creator3/1 -> pmac motor params/1
  Bus Creator5/1 -> hardware settings/1
  Bus Creator6/1 -> motor parameters/1
  Arm Shoulder Angle Offset/1 -> Bus Creator/1  "shoulder angle offset"
  Arm Elbow Angle Offset/1 -> Bus Creator/2  "elbow angle offset"
  Arm Shoulder X/1 -> Bus Creator/3  "Shoulder X"
  Arm Shoulder Y/1 -> Bus Creator/4  "Shoulder Y"
  Arm L1/1 -> Bus Creator/5  "L1"
  Arm L2/1 -> Bus Creator/6  "L2"
  Arm Pointer Offset/1 -> Bus Creator/7  "Pointer offset"
  Arm L3 Error/1 -> Bus Creator/8  "L3 Error"
  Bus Creator/1 -> calibration/1
  Bus Creator1/1 -> Bus Creator6/1, Bus Creator5/2, Bus Creator3/1  "R1"
  Arm robot version/1 -> Bus Creator6/3, Bus Creator5/3, decode robot/3(robot_version)  "robot version"
  [system_type] -> decode robot/1(system_type)
  decode robot/1(isEP) -> Bus Creator7/1  "isEP"
  decode robot/2(isHumanEXO) -> Bus Creator7/2  "isHumanExo"
  decode robot/3(isNHPEXO) -> Bus Creator7/3  "isNHPExo"
  decode robot/4(isClassicExo) -> Bus Creator7/4  "isClassicExo"
  decode robot/5(isUTSEXO) -> Bus Creator7/5  "isUTSExo"
  decode robot/6(isPMAC) -> Bus Creator7/6  "isPMAC"
  decode robot/7(isECAT) -> Bus Creator7/7  "isECAT"
  Bus Creator7/1 -> Bus Creator6/5  "R1Info"
  Status read1/1 -> Selector/1
  Selector/1 -> Bus Creator7/8  "robotRevision"

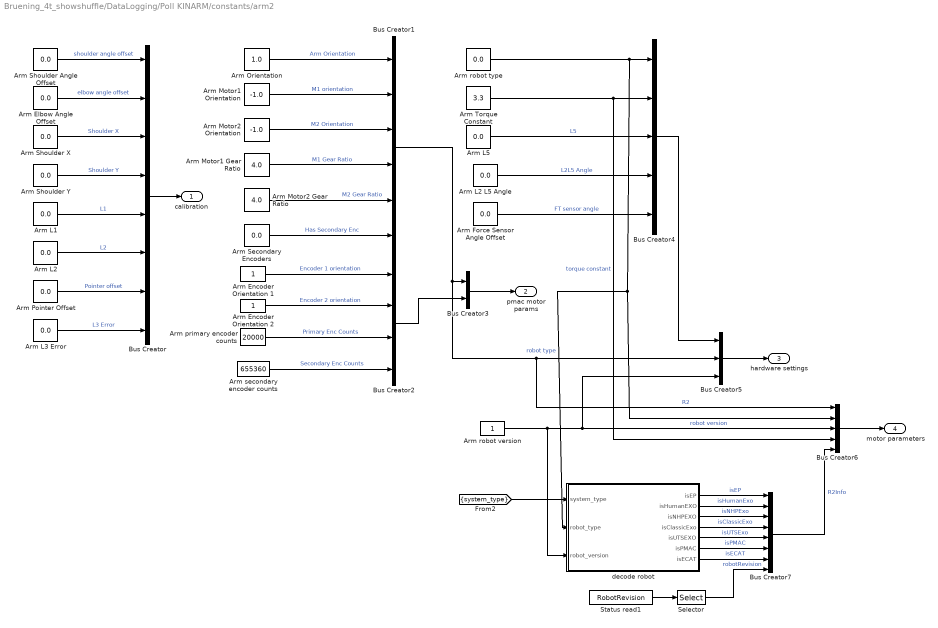
== system Bruening_4t_showshuffle/DataLogging/Poll KINARM/constants/arm2 ==
  Arm Elbow Angle Offset : Constant  Value=0.0
  Arm Encoder Orientation 1 : Constant
  Arm Encoder Orientation 2 : Constant
  Arm Force Sensor Angle Offset : Constant  Value=0.0
  Arm L1 : Constant  Value=0.0
  Arm L2 : Constant  Value=0.0
  Arm L2 L5 Angle : Constant  Value=0.0
  Arm L3 Error : Constant  Value=0.0
  Arm L5 : Constant  Value=0.0
  Arm Motor1 Gear Ratio : Constant  Value=4.0
  Arm Motor1 Orientation : Constant  Value=-1.0
  Arm Motor2 Gear Ratio : Constant  Value=4.0
  Arm Motor2 Orientation : Constant  Value=-1.0
  Arm Orientation : Constant  Value=1.0
  Arm Pointer Offset : Constant  Value=0.0
  Arm Secondary Encoders : Constant  Value=0.0
  Arm Shoulder Angle Offset : Constant  Value=0.0
  Arm Shoulder X : Constant  Value=0.0
  Arm Shoulder Y : Constant  Value=0.0
  Arm Torque Constant : Constant  Value=3.3
  Arm primary encoder counts : Constant  Value=20000
  Arm robot type : Constant  Value=0.0
  Arm robot version : Constant
  Arm secondary encoder counts : Constant  Value=655360
  Bus Creator : BusCreator  Inputs=8
  Bus Creator1 : BusCreator  Inputs=6
  Bus Creator2 : BusCreator
  Bus Creator3 : BusCreator  Inputs=2
  Bus Creator4 : BusCreator  Inputs=5
  Bus Creator5 : BusCreator  Inputs=3
  Bus Creator6 : BusCreator  Inputs=5
  Bus Creator7 : BusCreator  Inputs=8
  Selector : Selector  Indices=[2]
  Status read1 : DataStoreRead  DataStoreName=RobotRevision
  decode robot : MATLAB Function  TreatAsAtomicUnit=on
  calibration : Outport
  pmac motor params : Outport  Port=2
  hardware settings : Outport  Port=3
  motor parameters : Outport  Port=4
  wires:
  Arm secondary encoder counts/1 -> Bus Creator2/4  "Secondary Enc Counts"
  Arm primary encoder counts/1 -> Bus Creator2/3  "Primary Enc Counts"
  Arm Orientation/1 -> Bus Creator1/1  "Arm Orientation"
  Arm Motor1 Orientation/1 -> Bus Creator1/2  "M1 orientation"
  Arm Motor2 Orientation/1 -> Bus Creator1/3  "M2 Orientation"
  Arm Motor1 Gear Ratio/1 -> Bus Creator1/4  "M1 Gear Ratio"
  Arm Motor2 Gear Ratio/1 -> Bus Creator1/5  "M2 Gear Ratio"
  Arm Secondary Encoders/1 -> Bus Creator1/6  "Has Secondary Enc"
  Arm robot type/1 -> Bus Creator4/1, Bus Creator6/2, decode robot/2(robot_type)  "robot type"
  Arm Torque Constant/1 -> Bus Creator4/2, Bus Creator6/4  "torque constant"
  Arm L5/1 -> Bus Creator4/3  "L5"
  Arm L2 L5 Angle/1 -> Bus Creator4/4  "L2L5 Angle"
  Bus Creator4/1 -> Bus Creator5/1
  Arm Force Sensor Angle Offset/1 -> Bus Creator4/5  "FT sensor angle"
  Arm Encoder Orientation 1/1 -> Bus Creator2/1  "Encoder 1 orientation"
  Arm Encoder Orientation 2/1 -> Bus Creator2/2  "Encoder 2 orientation"
  Bus Creator2/1 -> Bus Creator3/2
  Bus Creator3/1 -> pmac motor params/1
  Bus Creator5/1 -> hardware settings/1
  Bus Creator6/1 -> motor parameters/1
  Arm Shoulder Angle Offset/1 -> Bus Creator/1  "shoulder angle offset"
  Arm Elbow Angle Offset/1 -> Bus Creator/2  "elbow angle offset"
  Arm Shoulder X/1 -> Bus Creator/3  "Shoulder X"
  Arm Shoulder Y/1 -> Bus Creator/4  "Shoulder Y"
  Arm L1/1 -> Bus Creator/5  "L1"
  Arm L2/1 -> Bus Creator/6  "L2"
  Arm Pointer Offset/1 -> Bus Creator/7  "Pointer offset"
  Arm L3 Error/1 -> Bus Creator/8  "L3 Error"
  Bus Creator/1 -> calibration/1
  Bus Creator1/1 -> Bus Creator6/1, Bus Creator5/2, Bus Creator3/1  "R2"
  Arm robot version/1 -> Bus Creator5/3, Bus Creator6/3, decode robot/3(robot_version)  "robot version"
  [system_type] -> decode robot/1(system_type)
  decode robot/1(isEP) -> Bus Creator7/1  "isEP"
  decode robot/2(isHumanEXO) -> Bus Creator7/2  "isHumanExo"
  decode robot/3(isNHPEXO) -> Bus Creator7/3  "isNHPExo"
  decode robot/4(isClassicExo) -> Bus Creator7/4  "isClassicExo"
  decode robot/5(isUTSEXO) -> Bus Creator7/5  "isUTSExo"
  decode robot/6(isPMAC) -> Bus Creator7/6  "isPMAC"
  decode robot/7(isECAT) -> Bus Creator7/7  "isECAT"
  Bus Creator7/1 -> Bus Creator6/5  "R2Info"
  Status read1/1 -> Selector/1
  Selector/1 -> Bus Creator7/8  "robotRevision"

== system Bruening_4t_showshuffle/DataLogging/Poll KINARM/constants/update constants subsystem ==
  Params : Inport
  Enable : EnablePort
  Arm Force Sensors : Constant  Value=[0 0]
  Bus Selector : BusSelector  OutputSignals=robot1 calibration params,robot2 calibration params
  Bus Selector1 : BusSelector  OutputSignals=robot1 hardware settings,robot2 hardware settings
  Bus to Vector{,1..3} (4 alike) : BusToVector
  Data Store Write : DataStoreWrite  DataStoreName=RobotCalibrations
  Data Store Write1 : DataStoreWrite  DataStoreName=HardwareSettings
  Data Store Write8 : DataStoreWrite  DataStoreName=ArmForceSensors
  Mux1 : Mux  Inputs=2
  Mux6 : Mux  Inputs=2
  wires:
  Mux6/1 -> Data Store Write/1
  Bus Selector/1 -> Bus to Vector/1  "<robot1 calibration params>"
  Bus Selector/2 -> Bus to Vector1/1  "<robot2 calibration params>"
  Mux1/1 -> Data Store Write1/1
  Params/1 -> Bus Selector1/1, Bus Selector/1
  Bus Selector1/1 -> Bus to Vector2/1  "<robot1 hardware settings>"
  Bus Selector1/2 -> Bus to Vector3/1  "<robot2 hardware settings>"
  Arm Force Sensors/1 -> Data Store Write8/1
  Bus to Vector/1 -> Mux6/1
  Bus to Vector1/1 -> Mux6/2
  Bus to Vector2/1 -> Mux1/1
  Bus to Vector3/1 -> Mux1/2

== system Bruening_4t_showshuffle/DataLogging/Poll KINARM/createKINData/hand feedback ==
  note: The hand feedback settings here may or may not be used by the hand
      | feedback block, depending on its block mask settings. They are
      | transferred to the hand feedback block via the KINdata data structure.
  Gaze Feedback Status : Constant  Value=0
  Hand Feedback Colour : Constant  Value=16777215
  Hand Feedback Feed Forward : Constant  Value=.03
  Hand Feedback Radius : Constant  Value=0.005
  Hand Feedback Source : Constant  Value=0
  Hand Feedback Status : Constant  Value=3
  Mux5 : Mux  Inputs=6
  hand feedback settings : Outport
  wires:
  Gaze Feedback Status/1 -> Mux5/6
  Hand Feedback Colour/1 -> Mux5/4
  Hand Feedback Status/1 -> Mux5/1
  Hand Feedback Source/1 -> Mux5/2
  Mux5/1 -> hand feedback settings/1
  Hand Feedback Feed Forward/1 -> Mux5/5
  Hand Feedback Radius/1 -> Mux5/3

== system Bruening_4t_showshuffle/DataLogging/Poll KINARM/Force Sensor Control/Force Sensor 1 Subsystem/If Action Subsystem ==
  In1 : Inport
  Enable : EnablePort
  Byte Reversal : xpcutilitieslib/Byte Reversal   numInp=1
  Byte Reversal1 : xpcutilitieslib/Byte Reversal   numInp=1
  Byte Reversal2 : xpcutilitieslib/Byte Reversal   numInp=1
  Constant : Constant  Value=4660  OutDataTypeStr=uint16
  Constant1 : Constant  Value=0  OutDataTypeStr=uint32
  Constant2 : Constant  Value=0  OutDataTypeStr=uint16
  Constant3 : Constant  Value=2  OutDataTypeStr=uint16
  Pack : xpcobsoletelib/Utilities/Pack   datatypes={'uint16', 'uint16', 'uint32'}  byteAlign=1
  Send : xpcrtudplib/Legacy UDP/Send   ipAddress=192.168.0.10  ipPort=49152  localPort=51000  vblLen=off  sampletime=-1
  Switch : Switch  Criteria=u2 > Threshold
  wires:
  In1/1 -> Switch/2
  Constant/1 -> Byte Reversal1/1
  Constant1/1 -> Byte Reversal2/1
  Constant3/1 -> Switch/1
  Constant2/1 -> Switch/3
  Switch/1 -> Byte Reversal/1
  Pack/1 -> Send/1
  Byte Reversal1/1 -> Pack/1
  Byte Reversal/1 -> Pack/2
  Byte Reversal2/1 -> Pack/3

== system Bruening_4t_showshuffle/DataLogging/Poll KINARM/Force Sensor Control/Force Sensor 2 Subsystem/Data Transfer Start Subsystem ==
  In2 : Inport
  Enable : EnablePort
  Byte Reversal : xpcutilitieslib/Byte Reversal   numInp=1
  Byte Reversal1 : xpcutilitieslib/Byte Reversal   numInp=1
  Byte Reversal2 : xpcutilitieslib/Byte Reversal   numInp=1
  Constant : Constant  Value=4660  OutDataTypeStr=uint16
  Constant1 : Constant  Value=0  OutDataTypeStr=uint32
  Constant2 : Constant  Value=0  OutDataTypeStr=uint16
  Constant3 : Constant  Value=2  OutDataTypeStr=uint16
  Pack : xpcobsoletelib/Utilities/Pack   datatypes={'uint16', 'uint16', 'uint32'}  byteAlign=1
  Send : xpcrtudplib/Legacy UDP/Send   ipAddress=192.168.0.11  ipPort=49152  localPort=51001  vblLen=off  sampletime=-1
  Switch : Switch  Criteria=u2 > Threshold
  wires:
  In2/1 -> Switch/2
  Constant/1 -> Byte Reversal1/1
  Constant1/1 -> Byte Reversal/1
  Constant3/1 -> Switch/1
  Constant2/1 -> Switch/3
  Switch/1 -> Byte Reversal2/1
  Pack/1 -> Send/1
  Byte Reversal/1 -> Pack/3
  Byte Reversal1/1 -> Pack/1
  Byte Reversal2/1 -> Pack/2

== system Bruening_4t_showshuffle/DataLogging/Poll KINARM/PMAC Subsystem/read_pmac/DPRAM Access Subsystem ==
  note: This PMAC needs a 16-bit integer for the watchdog input, but writemem
      | only writes singles.  So we need to typecast to single first
  note: This subsystem provides BKIN client software with access to the DPRAM of the motion control card.
      |
      | To read a value from DPRAM: write the value's offset to DPRAMReadOffset, set the switch indicating
      | whether the address holds a floating or fixed point value, then set the read switch high and allow the
      | result to propagate. Read the value, stored as a double, from DPRAMReadValue.
      |
      | To write a value to DPRAM: write the value to DPRAMWriteValue and its offset to DPRAMWriteOffset,
      | set the write switch high, and then allow the result to propagate. There is currently no option to write
      | values as UInt32s, akin to that for reading values.
      |
      | The default value for the offsets (0x216) is the lowest meaningful offset, the PLC switch variable.
  Counter Free-Running : simulink/Sources/Counter Free-Running  NumBits=16  tsamp=-1
  DPRAM Read Offset : Constant  Value=534  OutDataTypeStr=double
  DPRAM Read Value : Gain  SaturateOnIntegerOverflow=on  OutDataTypeStr=Inherit: Same as input  ParamDataTypeStr=Inherit: Same as input
  DPRAM WatchDog offset : Constant  Value=627  OutDataTypeStr=double
  DPRAM Write Offset : Constant  Value=534  OutDataTypeStr=double
  DPRAM Write Value : Constant
  Data Type Conversion : DataTypeConversion  OutDataTypeStr=uint32  SaturateOnIntegerOverflow=on  RndMeth=Zero
  If : If  NumInputs=2  IfExpression=u2 > u1  ShowElse=off
  If1 : If  NumInputs=2  IfExpression=u2 > u1  ShowElse=off
  Read DPRAM : Subsystem  TreatAsAtomicUnit=on
  Read Switch : Constant  Value=0
  Read as UInt32 : Constant  Value=0  OutDataTypeStr=double
  Terminator : Terminator
  TypeCast : MATLAB Function  TreatAsAtomicUnit=on
  Unit Delay : UnitDelay  SampleTime=-1
  Unit Delay1 : UnitDelay  SampleTime=-1
  Write : S-Function  Priority=6  FunctionName=mcc_writemem
  Write DPRAM : Subsystem  TreatAsAtomicUnit=on
  Write Switch : Constant  Value=0
  wires:
  TypeCast/1(y) -> Write/2
  DPRAM Write Offset/1 -> Write DPRAM/1(offset)
  DPRAM Write Value/1 -> Write DPRAM/2(value)
  If1/1 -> Write DPRAM/Action
  Write Switch/1 -> Unit Delay1/1, If1/2
  DPRAM Read Value/1 -> Terminator/1
  Read DPRAM/1(result) -> DPRAM Read Value/1
  If/1 -> Read DPRAM/Action
  DPRAM Read Offset/1 -> Read DPRAM/1(offset)
  Read Switch/1 -> Unit Delay/1, If/2
  Unit Delay/1 -> If/1
  Unit Delay1/1 -> If1/1
  Read as UInt32/1 -> Read DPRAM/2(read as uint32)
  Data Type Conversion/1 -> Write/1
  DPRAM WatchDog offset/1 -> Data Type Conversion/1
  Counter Free-Running/1 -> TypeCast/1(u)

== system Bruening_4t_showshuffle/DataLogging/Poll KINARM/PMAC Subsystem/read_pmac/DPRAM Access Subsystem/Read DPRAM ==
  offset : Inport
  read as uint32 : Inport  Port=2
  Action Port : ActionPort  ActionType=then
  Data Type Conversion : DataTypeConversion  OutDataTypeStr=uint32  SaturateOnIntegerOverflow=on  RndMeth=Zero
  Data Type Conversion1 : DataTypeConversion  OutDataTypeStr=double  SaturateOnIntegerOverflow=on  RndMeth=Zero
  Data Type Conversion2 : DataTypeConversion  OutDataTypeStr=uint32  SaturateOnIntegerOverflow=on  RndMeth=Zero
  Mux : Mux  Inputs=2
  Read : S-Function  Priority=6  FunctionName=mcc_readmem
  result : Outport
  wires:
  Data Type Conversion/1 -> Mux/1
  Data Type Conversion1/1 -> result/1
  Read/1 -> Data Type Conversion1/1
  offset/1 -> Data Type Conversion/1
  read as uint32/1 -> Data Type Conversion2/1
  Data Type Conversion2/1 -> Mux/2
  Mux/1 -> Read/1

== system Bruening_4t_showshuffle/DataLogging/Poll KINARM/PMAC Subsystem/read_pmac/DPRAM Access Subsystem/Write DPRAM ==
  offset : Inport
  value : Inport  Port=2
  Action Port : ActionPort  ActionType=then
  Data Type Conversion : DataTypeConversion  OutDataTypeStr=uint32  SaturateOnIntegerOverflow=on  RndMeth=Zero
  Data Type Conversion1 : DataTypeConversion  OutDataTypeStr=single  SaturateOnIntegerOverflow=on  RndMeth=Zero
  Write : S-Function  Priority=6  FunctionName=mcc_writemem
  wires:
  Data Type Conversion1/1 -> Write/2
  Data Type Conversion/1 -> Write/1
  offset/1 -> Data Type Conversion/1
  value/1 -> Data Type Conversion1/1
